simulink model "blade_transfer_function_comparison"  (R2022a)
settings: Solver=VariableStepAuto  StartTime=0.0  StopTime=10  RelTol=1e-3
undefined symbols (not defined in the file or in its folder): actuator_fast, actuator_nominal, actuator_slow
settings Model: Creator=Niccolò  LastModifiedBy=Niccolò

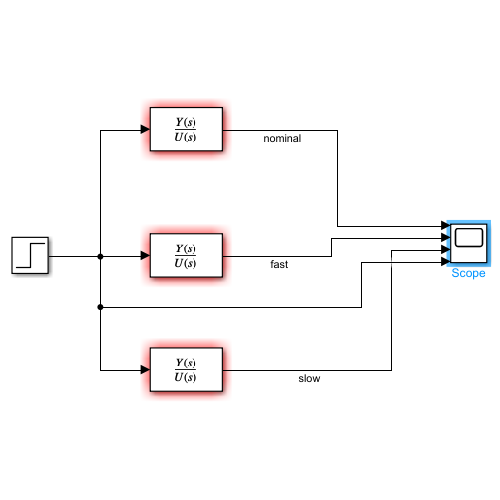
[thumbnail: Simulink's stored preview of the top-level diagram]
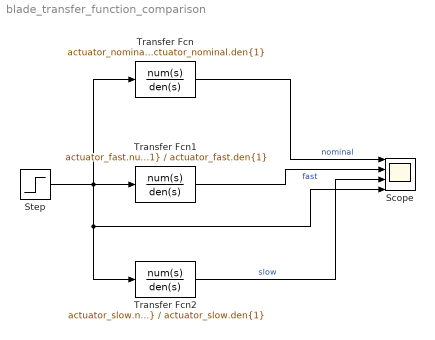
== system blade_transfer_function_comparison ==
  Scope : Scope  NumInputPorts=4
  Step : Step  Time=0.5  SampleTime=0
  Transfer Fcn : TransferFcn  Numerator=actuator_nominal.num{1}  Denominator=actuator_nominal.den{1}
  Transfer Fcn1 : TransferFcn  Numerator=actuator_fast.num{1}  Denominator=actuator_fast.den{1}
  Transfer Fcn2 : TransferFcn  Numerator=actuator_slow.num{1}  Denominator=actuator_slow.den{1}
  wires:
  Transfer Fcn/1 -> Scope/1  "nominal"
  Transfer Fcn1/1 -> Scope/2  "fast"
  Transfer Fcn2/1 -> Scope/3  "slow"
  Step/1 -> Transfer Fcn/1, Transfer Fcn1/1, Transfer Fcn2/1, Scope/4
